simulink model "solor_model"  (R2015a)
settings: Solver=ode45  StartTime=0.0  StopTime=10.0  RelTol=1e-3
InitFcn:
  | load pr
StartFcn:
  | load pr
values from neighbouring files (symbols this model uses):
  opt = 75    [pr.mat]    (also in solor_irra_var.m = 30; solor_temp_var.m = temp(i))
  srad = 500    [pr.mat]    (also in solor_irra_var.m = srd(i); solor_temp_var.m)
libraries: simulink x2, powerlib x1
settings Model: Creator=Rajora  LastModifiedBy=Pro. Shrikant
settings DataIOCC: SignalLoggingSaveFormat=ModelDataLogs
settings OptimizationCC: ExpressionDepthLimit=2147483647
settings DebuggingCC: UnderspecifiedInitializationDetection=Classic  MergeDetectMultiDrivingBlocksExec=none  SolverPrmCheckMsg=warning  FcnCallInpInsideContextMsg=EnableAllAsWarning  StateNameClashWarn=warning

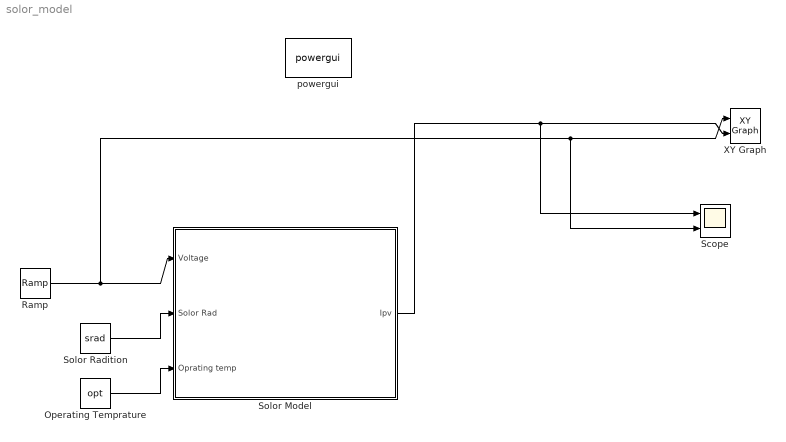
== system solor_model ==
  Operating Temprature : Constant  Value=opt
  Ramp : simulink/Sources/Ramp  slope=3  start=0  X0=0
  Scope : Scope  NumInputPorts=2
      settings: YMin=-5~-5  YMax=5~5
  Solor Model : Subsystem
  Solor Radition : Constant  Value=srad
  XY Graph : simulink/Sinks/XY Graph  xmin=-1  xmax=22  ymin=-1  ymax=10  st=-1
  powergui : powerlib/powergui  Priority=1  SimulationMode=Discrete  SolverType=Tustin  SampleTime=1e-6  frequency=60  SPID=off  DisableSnubberDevices=off  DisableRonSwitches=off  DisableVfSwitches=off  SwTol=0  DisplayEquations=off  Interpol=off  methode=off  Ts=0  FunctionMessages=off  echomessages=off  HookPort=off  EnableUseOfTLC=off  x0status=blocks  frequencyindice=0  Pbase=100e6  ErrMax=1e-4  Iterations=50  UnitsV=kV  UnitsW=MW  buscounter=0  RestoreLinks=warning  ResistiveCurrentMeasurement=off  Frange=[0:2:500]  Ylog=off  Xlog=on  ShowGrid=off  save=off  variable=ZData  structure=0  ZoomFFT=off  StartTime=0.0  cycles=1  DisplayStyle=1  fundamental=60  FreqAxis=off  MaxFrequency=1000  frequencyindicesteady=1  RmsSteady=1  display=off
  wires:
  Operating Temprature/1 -> Solor Model/3(Oprating temp)
  Solor Radition/1 -> Solor Model/2(Solor Rad)
  Solor Model/1(Ipv) -> XY Graph/2, Scope/1
  Ramp/1 -> Solor Model/1(Voltage), XY Graph/1, Scope/2

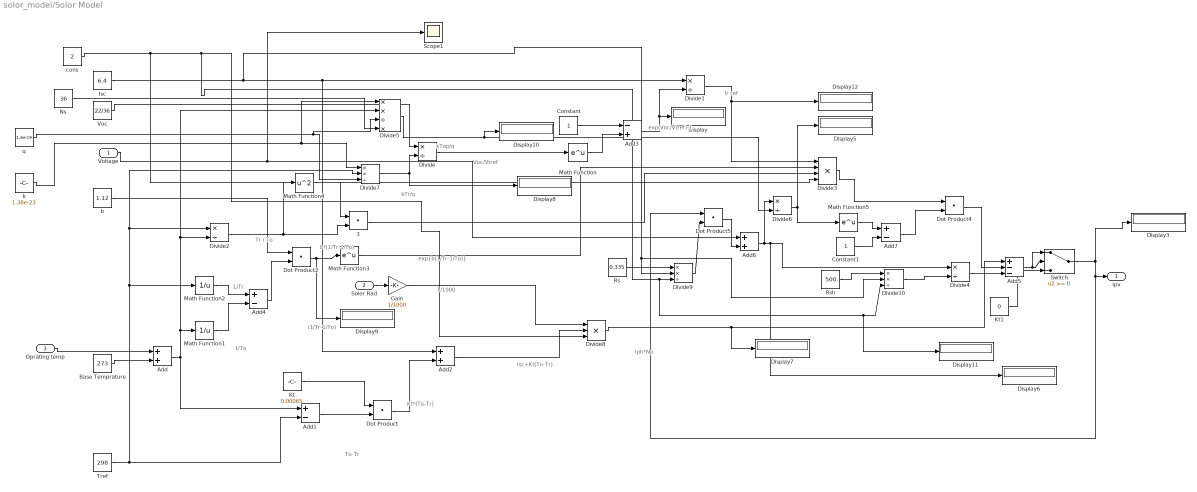
== system solor_model/Solor Model ==
  note: Tr / To
  note: kTop/q
  note: 1/Tr
  note: 1/To
  note: (1/Tr-1/To)
  note: b*(1/Tr-1/To)
  note: exp{b(1/Tr-1/To)}
  note: To-Tr
  note: Kt*(To-Tr)
  note: Isc+Kt(To-Tr)
  note: 1/1000
  note: Iph*Np
  note: kTr/q
  note: Voc/Vtref
  note: exp(Voc/Vtref)-1
  note: Ir ref
  Voltage : Inport
  Solor Rad : Inport  Port=2
  Oprating temp : Inport  Port=3
  3 : DotProduct  InputSameDT=on  OutDataTypeStr=Inherit: Inherit via internal rule
  Add : Sum
  Add1 : Sum  Inputs=+-
  Add2 : Sum
  Add3 : Sum  Inputs=-+
  Add4 : Sum  Inputs=+-
  Add5 : Sum  Inputs=+--
  Add6 : Sum
  Add7 : Sum  Inputs=+-
  Base Temprature : Constant  Value=273
  Constant : Constant
  Constant1 : Constant
  Display{,3,5..12} (10 alike) : Display
  Divide{,1..2,4,6} (5 alike) : Product  Inputs=*/
  Divide10 : Product  Inputs=**/
  Divide3 : Product  Inputs=****
  Divide5 : Product  Inputs=**/*
  Divide7 : Product  Inputs=**/
  Divide8 : Product  Inputs=***
  Divide9 : Product  Inputs=**/
  Dot Product{,2,4..5} (4 alike) : DotProduct  InputSameDT=on  OutDataTypeStr=Inherit: Inherit via internal rule
  Gain : Gain  Gain=1/1000
  Isc : Constant  Value=6.4
  Kt : Constant  Value=0.00065
  Kt1 : Constant  Value=0
  Math Function : Math  SaturateOnIntegerOverflow=on
  Math Function1 : Math  Operator=reciprocal  SaturateOnIntegerOverflow=on
  Math Function2 : Math  Operator=reciprocal  SaturateOnIntegerOverflow=on
  Math Function3 : Math  SaturateOnIntegerOverflow=on
  Math Function4 : Math  Operator=square  SaturateOnIntegerOverflow=on
  Math Function5 : Math  SaturateOnIntegerOverflow=on
  Ns : Constant  Value=36
  Rs : Constant  Value=0.335
  Rsh : Constant  Value=500
  Scope1 : Scope
  Switch : Switch
  Tref : Constant  Value=298
  Voc : Constant  Value=22/36
  b : Constant  Value=1.12
  cons : Constant  Value=2
  k : Constant  Value=1.38e-23
  q : Constant  Value=1.6e-19
  Ipv : Outport
  wires:
  Base Temprature/1 -> Add/2
  Add1/1 -> Dot Product/2
  Kt/1 -> Dot Product/1
  Dot Product/1 -> Add2/2
  Isc/1 -> Add2/1, Divide1/1, Divide9/2, Divide10/2
  Add2/1 -> Divide8/2
  Gain/1 -> Divide8/1
  Divide8/1 -> Add5/1, Display7/1
  Voltage/1 -> Add6/1, Scope1/1
  Voc/1 -> Divide/1
  Divide/1 -> Math Function/1
  Math Function/1 -> Add3/2
  Add3/1 -> Divide1/2, Display/1
  Math Function2/1 -> Add4/1
  Math Function1/1 -> Add4/2
  Add4/1 -> Dot Product2/2
  b/1 -> Dot Product2/1
  Dot Product2/1 -> Math Function3/1, Display9/1
  Math Function3/1 -> Divide3/2
  Math Function4/1 -> 3/1
  Divide2/1 -> 3/2, Math Function4/1
  Divide1/1 -> Divide3/1, Display12/1
  3/1 -> Divide3/3
  Divide3/1 -> Dot Product4/1
  Dot Product4/1 -> Add5/2
  Dot Product5/1 -> Add6/2
  Add6/1 -> Divide4/1, Display6/1, Divide6/1
  Divide4/1 -> Add5/3
  q/1 -> Divide5/3, Divide7/3
  Divide5/1 -> Divide6/2, Display10/1
  Constant1/1 -> Add7/2
  Add7/1 -> Dot Product4/2
  Math Function5/1 -> Add7/1
  Divide6/1 -> Math Function5/1, Display5/1
  Add5/1 -> Switch/2, Switch/1
  Switch/1 -> Dot Product5/1, Ipv/1, Display3/1
  Divide7/1 -> Divide/2, Display8/1
  Tref/1 -> Math Function2/1, Divide2/1, Divide7/2, Add1/2
  Constant/1 -> Add3/1
  Ns/1 -> Divide5/4
  cons/1 -> Divide3/4, Divide8/3, Divide9/3, Divide10/3, Display11/1
  Rs/1 -> Divide9/1
  Divide9/1 -> Dot Product5/2
  Rsh/1 -> Divide10/1
  Divide10/1 -> Divide4/2
  k/1 -> Divide5/1, Divide7/1
  Add/1 -> Math Function1/1, Divide2/2, Divide5/2, Add1/1
  Kt1/1 -> Switch/3
  Solor Rad/1 -> Gain/1
  Oprating temp/1 -> Add/1
